simulink model "state_estim_mdl_2023a"  (R2023a)
settings: Solver=VariableStepAuto  StartTime=0.0  StopTime=20  RelTol=1e-3
values from neighbouring files (symbols this model uses):
  ic = 0    [state_estim.m]
  L = acker(transpose(Ae), transpose(Ce), -2 * [1, 1, 1, 1, 1])    [state_estim.m]
  T = 1e-3    (= 0.001)    [state_estim.m]
undefined symbols (not defined in the file or in its folder): umax
libraries: simulink x2
settings Model: Creator=rapaja  LastModifiedBy=Predrag
settings SolverCC: AlgebraicLoopSolver=TrustRegion
settings DebuggingCC: UnconnectedInputMsg=warning  UnconnectedOutputMsg=warning  UnconnectedLineMsg=warning
settings ModelReferenceCC: EnableRefExpFcnMdlSchedulingChecks=on
settings ConfigComp: CovBoundaryAbsTol=1.0e-5

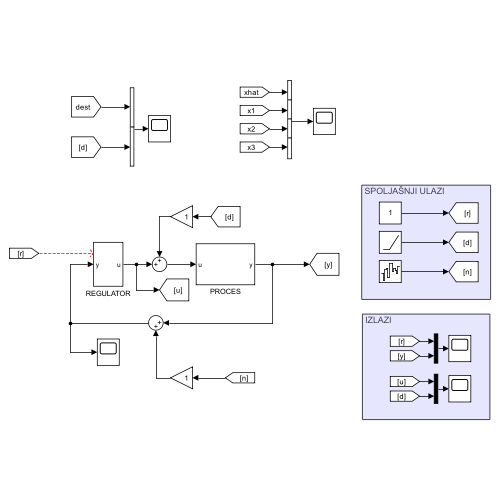
[thumbnail: Simulink's stored preview of the top-level diagram]
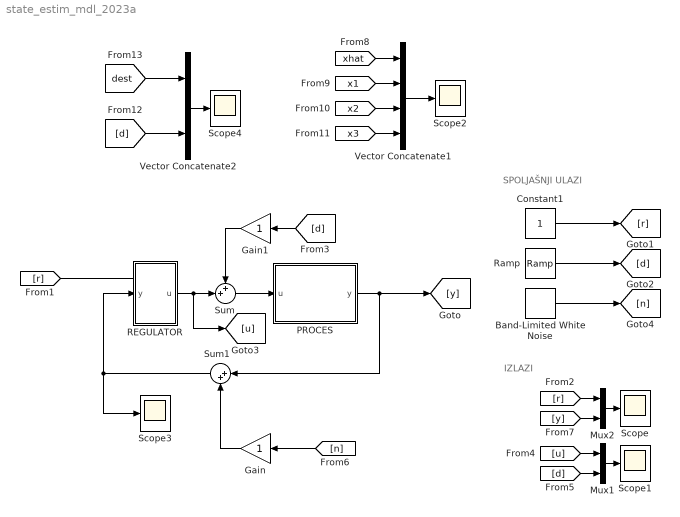
== system state_estim_mdl_2023a ==
  note: IZLAZI
  note: SPOLJAŠNJI ULAZI
  Band-Limited White Noise : simulink/Sources/Band-Limited White Noise  Cov=[0.00001]  Ts=T  seed=[23341]
  Constant1 : Constant
  Gain : Gain
  Gain1 : Gain
  Mux1 : Mux  Inputs=2
  Mux2 : Mux  Inputs=2
  PROCES : Subsystem
  REGULATOR : Subsystem
  Ramp : simulink/Sources/Ramp  slope=1  start=1  InitialOutput=2
  Scope{,1..4} (5 alike) : Scope
  Sum : Sum  Inputs=++|
  Sum1 : Sum  Inputs=|++
  Vector Concatenate1 : Concatenate  NumInputs=4
  Vector Concatenate2 : Concatenate
  wires:
  REGULATOR/1(u) -> Sum/2, [u]
  [d] -> Gain1/1
  Band-Limited White Noise/1 -> [n]
  Gain/1 -> Sum1/2
  Gain1/1 -> Sum/1
  Ramp/1 -> [d]
  [r] -> Mux2/1
  [y] -> Mux2/2
  Mux2/1 -> Scope/1
  Mux1/1 -> Scope1/1
  [u] -> Mux1/1
  [d] -> Mux1/2
  PROCES/1(y) -> Sum1/1, [y]
  [r] -> ?
  Sum/1 -> PROCES/1(u)
  Sum1/1 -> Scope3/1, REGULATOR/1(y)
  Constant1/1 -> [r]
  Vector Concatenate1/1 -> Scope2/1
  [xhat] -> Vector Concatenate1/1
  [x3] -> Vector Concatenate1/4
  [x2] -> Vector Concatenate1/3
  [x1] -> Vector Concatenate1/2
  [n] -> Gain/1
  Vector Concatenate2/1 -> Scope4/1
  [d] -> Vector Concatenate2/2
  [dest] -> Vector Concatenate2/1

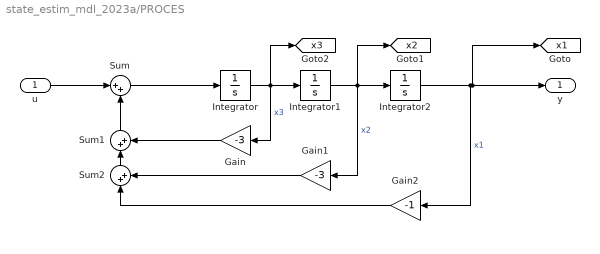
== system state_estim_mdl_2023a/PROCES ==
  u : Inport
  Gain : Gain  Gain=-3
  Gain1 : Gain  Gain=-3
  Gain2 : Gain  Gain=-1
  Integrator : Integrator  InitialCondition=ic
  Integrator1 : Integrator  InitialCondition=ic
  Integrator2 : Integrator  InitialCondition=ic
  Sum : Sum  Inputs=|++
  Sum1 : Sum  Inputs=|++
  Sum2 : Sum  Inputs=|++
  y : Outport
  tag scope: x1=global, x2=global, x3=global
  wires:
  Integrator2/1 -> [x1], y/1, Gain2/1  "x1"
  Integrator1/1 -> [x2], Integrator2/1, Gain1/1  "x2"
  Integrator/1 -> [x3], Integrator1/1, Gain/1  "x3"
  u/1 -> Sum/1
  Sum/1 -> Integrator/1
  Gain/1 -> Sum1/2
  Sum1/1 -> Sum/2
  Sum2/1 -> Sum1/1
  Gain1/1 -> Sum2/2
  Gain2/1 -> Sum2/1

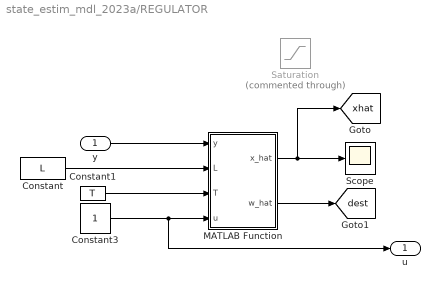
== system state_estim_mdl_2023a/REGULATOR ==
  y : Inport
  Constant : Constant  Value=L  VectorParams1D=off
  Constant1 : Constant  Value=T
  Constant3 : Constant
  MATLAB Function : MATLAB Function  TreatAsAtomicUnit=on
  Saturation : Saturate  Commented=through  UpperLimit=umax  LowerLimit=-umax
  Scope : Scope
  u : Outport
  tag scope: dest=global, xhat=global
  wires:
  y/1 -> MATLAB Function/1(y)
  Constant/1 -> MATLAB Function/2(L)
  Constant1/1 -> MATLAB Function/3(T)
  Constant3/1 -> u/1, MATLAB Function/4(u)
  MATLAB Function/1(x_hat) -> [xhat], Scope/1
  MATLAB Function/2(w_hat) -> [dest]

== matlab function state_estim_mdl_2023a/REGULATOR/MATLAB Function ==
  settings: updateMethod=DISCRETE  sampleTime=T
  data: y input; x_hat output; L input; T input; u input; w_hat output
function [x_hat, w_hat] = fcn(y, L, T, u)
persistent x1hat
persistent x2hat
persistent x3hat
persistent w1hat
persistent w2hat

if(isempty(x1hat))
    x1hat = 0;
end
if(isempty(x2hat))
    x2hat = 0;
end
if(isempty(x3hat))
    x3hat = 0;
end
if(isempty(w1hat))
    w1hat = 0;
end
if(isempty(w2hat))
    w2hat = 0;
end
e = y - x1hat;

x1hat_n = x1hat + T * (x2hat + L(1, 1) * e);
x2hat_n = x2hat + T * (x3hat + L(1, 2) * e);
x3hat_n = x3hat + T * (-3*x3hat - 3*x2hat -x1hat + u + w1hat + L(1, 3) * e);
w1hat_n = w1hat + T * ( w2hat + L(1, 4) * e);
w2hat_n = w2hat + T * (L(1, 5) * e);

x1hat = x1hat_n;
x2hat = x2hat_n;
x3hat = x3hat_n;
w1hat = w1hat_n;
w2hat = w2hat_n;

x_hat = [x1hat, x2hat, x3hat];
w_hat = w1hat;
